simulink model "Project3_MODEL"  (R2023b)
settings: Solver=FixedStepAuto  StartTime=0.0  StopTime=765  FixedStep=0.001  RelTol=1e-3
values from neighbouring files (symbols this model uses):
  DriveData = [0 ... (first row only)    [initHighwayCycle.m]    (also in initUrbanCycle.m)
  mph2mps = 1600/3600    (= 0.444444444444)    [Project3_init.m]
  Time = (0:1:765)'    [initHighwayCycle.m]    (also in initUrbanCycle.m = (0:1:1369)')
undefined symbols (not defined in the file or in its folder): batData, carData, motorData
libraries: slpidlib x1
settings Model: Creator=anshu16  LastModifiedBy=turtl
settings OptimizationCC: ReuseModelBlockBuffer=off
settings DebuggingCC: UnconnectedInputMsg=warning  UnconnectedOutputMsg=warning  UnconnectedLineMsg=warning
settings ModelReferenceCC: EnableRefExpFcnMdlSchedulingChecks=on
settings SFSimCC: CustomCodeUndefinedFunction=UseInterfaceOnly

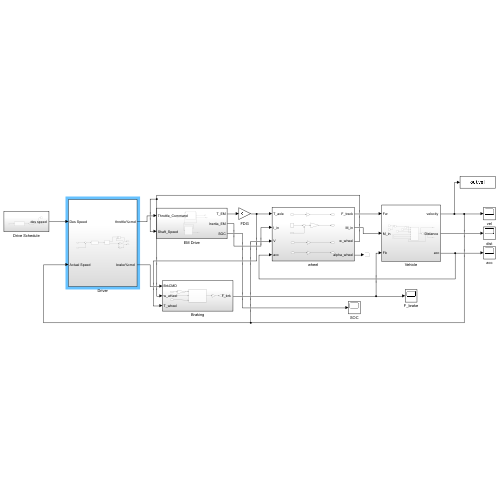
[thumbnail: Simulink's stored preview of the top-level diagram]
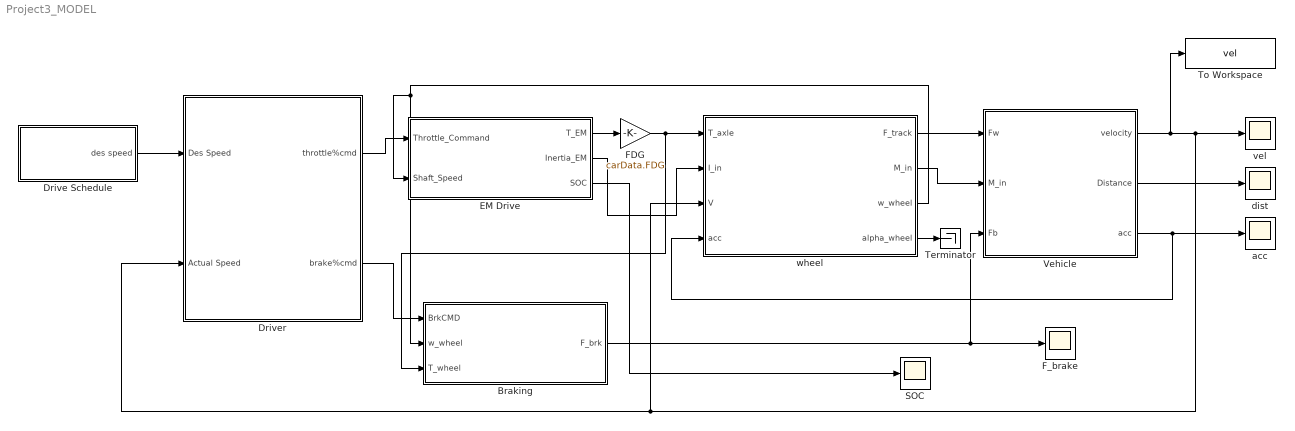
== system Project3_MODEL ==
  Braking : Subsystem
  Drive Schedule : Subsystem
  "Driver " : Subsystem
  EM Drive : Subsystem
  FDG : Gain  Gain=carData.FDG
  F_brake : Scope
  SOC : Scope
  Terminator : Terminator
  To Workspace : ToWorkspace  VariableName=vel  SaveFormat=Timeseries  SampleTime=-1
  Vehicle : Subsystem
  acc : Scope
  dist : Scope
  vel : Scope
  "wheel " : Subsystem
  wires:
  Drive Schedule/1("des speed ") -> "Driver "/1("Des Speed ")
  "Driver "/2("brake%cmd ") -> Braking/1("BrkCMD ")
  Braking/1("F_brk ") -> Vehicle/3("Fb "), F_brake/1
  Vehicle/3(acc) -> acc/1, "wheel "/4(acc)
  FDG/1 -> Braking/3(T_wheel), "wheel "/1(T_axle)
  EM Drive/2(Inertia_EM) -> "wheel "/2(I_in)
  "wheel "/2(M_in) -> Vehicle/2("M_in ")
  "wheel "/1(F_track) -> Vehicle/1("Fw ")
  Vehicle/2("Distance ") -> dist/1
  Vehicle/1("velocity ") -> To Workspace/1, vel/1, "wheel "/3(V), "Driver "/2(Actual Speed)
  "wheel "/4(alpha_wheel) -> Terminator/1
  "wheel "/3(w_wheel) -> Braking/2("w_wheel "), EM Drive/2(Shaft_Speed)
  "Driver "/1(throttle%cmd) -> EM Drive/1(Throttle_Command)
  EM Drive/3(SOC) -> SOC/1
  EM Drive/1(T_EM) -> FDG/1

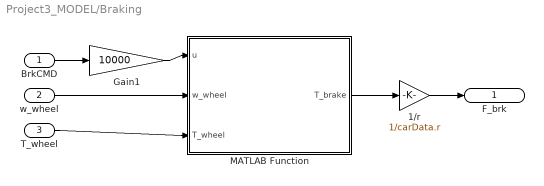
== system Project3_MODEL/Braking ==
  "BrkCMD " : Inport
  "w_wheel " : Inport  Port=2
  T_wheel : Inport  Port=3
  1/r : Gain  Gain=1/carData.r
  Gain1 : Gain  Gain=10000
  MATLAB Function : MATLAB Function  TreatAsAtomicUnit=on
  "F_brk " : Outport  VectorParamsAs1DForOutWhenUnconnected=off
  wires:
  "BrkCMD "/1 -> Gain1/1
  Gain1/1 -> MATLAB Function/1(u)
  MATLAB Function/1(T_brake) -> 1/r/1
  "w_wheel "/1 -> MATLAB Function/2(w_wheel)
  T_wheel/1 -> MATLAB Function/3(T_wheel)
  1/r/1 -> "F_brk "/1

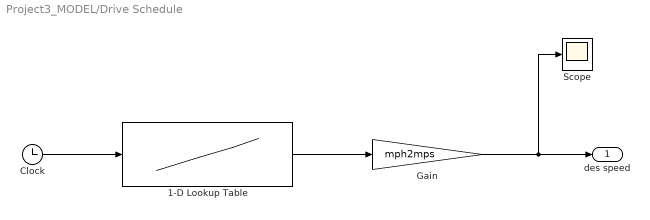
== system Project3_MODEL/Drive Schedule ==
  1-D Lookup Table : Lookup_n-D  NumberOfTableDimensions=1  BreakpointsForDimension1=Time  Table=DriveData  InternalRulePriority=Speed  RndMeth=Simplest
  Clock : Clock
  Gain : Gain  Gain=mph2mps
  Scope : Scope
  "des speed " : Outport  VectorParamsAs1DForOutWhenUnconnected=off
  wires:
  Clock/1 -> 1-D Lookup Table/1
  1-D Lookup Table/1 -> Gain/1
  Gain/1 -> "des speed "/1, Scope/1

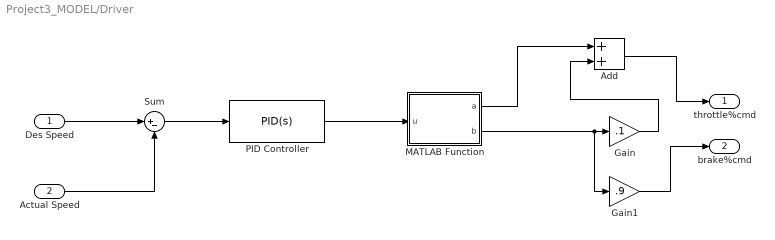
== system Project3_MODEL/Driver  ==
  "Des Speed " : Inport
  Actual Speed : Inport  Port=2
  Add : Sum
  Gain : Gain  Gain=.1
  Gain1 : Gain  Gain=.9
  MATLAB Function : MATLAB Function  TreatAsAtomicUnit=on
  PID Controller : slpidlib/PID Controller  Controller=PID  Form=Parallel  TimeDomain=Continuous-time  UseExternalTs=off  SampleTime=-1  IntegratorMethod=Forward Euler  FilterMethod=Forward Euler  ControllerParametersSource=internal  P=2.5  I=.1  UseKiTs=off  D=.5  N=100  UseFilter=on  TunerSelectOption=Transfer Function Based (PID Tuner App)  InitialConditionSource=internal  InitialConditionForIntegrator=0  InitialConditionForFilter=0  DifferentiatorICPrevScaledInput=0  ExternalReset=none  TrackingMode=off  Kt=1  LimitOutput=on  SatLimitsSource=internal  UpperSaturationLimit=1  LowerSaturationLimit=-1  LinearizeAsGain=off  AntiWindupMode=none  Kb=1  LimitIntegrator=off  UpperIntegratorSaturationLimit=inf  LowerIntegratorSaturationLimit=-inf  POutMin=[]  POutMax=[]  IOutMin=[]  IOutMax=[]  DOutMin=[]  DOutMax=[]  NOutMin=[]  NOutMax=[]  SumOutMin=[]  SumOutMax=[]  SaturationOutMin=[]  SaturationOutMax=[]  PParamMin=[]  PParamMax=[]  IParamMin=[]  IParamMax=[]  DParamMin=[]  DParamMax=[]  NParamMin=[]  NParamMax=[]  KbParamMin=[]  KbParamMax=[]  KtParamMin=[]  KtParamMax=[]  KbOutMin=[]  KbOutMax=[]  KtOutMin=[]  KtOutMax=[]  IntegratorOutMin=[]  IntegratorOutMax=[]  FilterOutMin=[]  FilterOutMax=[]  SumI1OutMin=[]  SumI1OutMax=[]  SumI2OutMin=[]  SumI2OutMax=[]  SumI3OutMin=[]  SumI3OutMax=[]  SumI4OutMin=[]  SumI4OutMax=[]  SumDOutMin=[]  SumDOutMax=[]  DifferentiatorOutMin=[]  DifferentiatorOutMax=[]  FilterDiffOutCoefMin=[]  FilterDiffOutCoefMax=[]  ReciprocalOutMin=[]  ReciprocalOutMax=[]  SumDenOutMin=[]  SumDenOutMax=[]  SumNumOutMin=[]  SumNumOutMax=[]  DivideOutMin=[]  DivideOutMax=[]  UdiffTsProdOutMin=[]  UdiffTsProdOutMax=[]  NTsProdOutMin=[]  NTsProdOutMax=[]  UintegralTsProdOutMin=[]  UintegralTsProdOutMax=[]  UngainTsProdOutMin=[]  UngainTsProdOutMax=[]  ClampingZeroOutDataTypeStr=Inherit: Inherit via back propagation  ClampingZeroOutMin=[]  ClampingZeroOutMax=[]  FilterDenConstantOutDataTypeStr=Inherit: Inherit via back propagation  FilterDenConstantOutMin=[]  FilterDenConstantOutMax=[]  PCopyOutDataTypeStr=Inherit: Inherit via back propagation  PCopyOutMin=[]  PCopyOutMax=[]  NCopyOutDataTypeStr=Inherit: Inherit via back propagation  NCopyOutMin=[]  NCopyOutMax=[]  IntegratorContinuousStateAttributes=''  IntegratorStateMustResolveToSignalObject=off  IntegratorRTWStateStorageClass=Auto  FilterContinuousStateAttributes=''  FilterStateMustResolveToSignalObject=off  FilterRTWStateStorageClass=Auto  ParallelPVariant=InternalParameters  IdealPVariant=Disabled  IVariant=InternalParameters  DVariant=InternalParameters  IntegratorVariant=Continuous  SatVariant=Enabled  AWVariant=Passthrough  PCopyVariant=Disabled  TRVariant=Disabled  FdbkBlocksVariant=Forward  IdealPFdbkVariant=Disabled  SatFdbkVariant=Disabled  DerivativeFilterVariant=ContFilter  NVariant=InternalParameters  NCopyVariant=Disabled  FilterICVariant=InternalICsFilter  IntegratorICVariant=InternalICs  ExternalResetVariant=Disabled  TRSumVariant=Passthrough  SumFdbkVariant=Disabled  SumVariant=Sum_PID  TsampFilterVariant=InternalTs  TsampNgainVariant=Passthrough  TsampIntegralVariant=Disabled_SignalSpec  ExternalSaturationOutDataTypeStr=Inherit: Same as second input
  Sum : Sum  Inputs=|+-
  throttle%cmd : Outport
  "brake%cmd " : Outport  Port=2
  wires:
  "Des Speed "/1 -> Sum/1
  Actual Speed/1 -> Sum/2
  Sum/1 -> PID Controller/1
  PID Controller/1 -> MATLAB Function/1(u)
  Gain/1 -> Add/2
  MATLAB Function/2(b) -> Gain/1, Gain1/1
  MATLAB Function/1(a) -> Add/1
  Add/1 -> throttle%cmd/1
  Gain1/1 -> "brake%cmd "/1

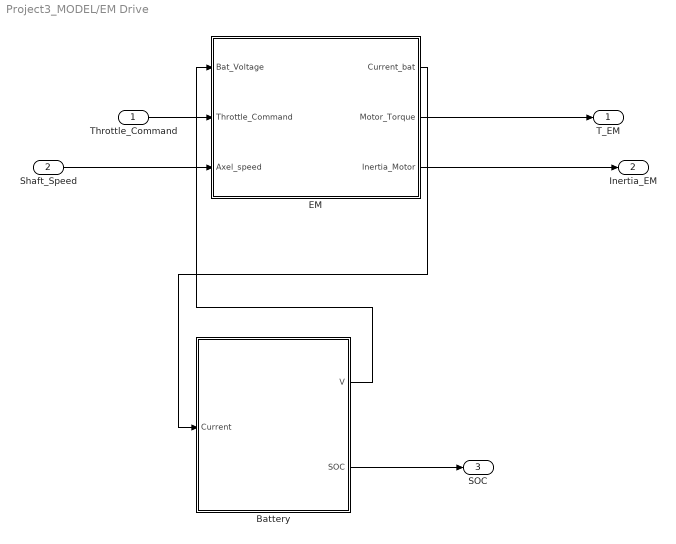
== system Project3_MODEL/EM Drive ==
  Throttle_Command : Inport
  Shaft_Speed : Inport  Port=2
  Battery : Subsystem
  EM : Subsystem
  T_EM : Outport
  Inertia_EM : Outport  Port=2
  SOC : Outport  Port=3
  wires:
  EM/1(Current_bat) -> Battery/1(Current)
  Throttle_Command/1 -> EM/2(Throttle_Command)
  Shaft_Speed/1 -> EM/3(Axel_speed)
  EM/2(Motor_Torque) -> T_EM/1
  EM/3(Inertia_Motor) -> Inertia_EM/1
  Battery/1(V) -> EM/1(Bat_Voltage)
  Battery/2(SOC) -> SOC/1

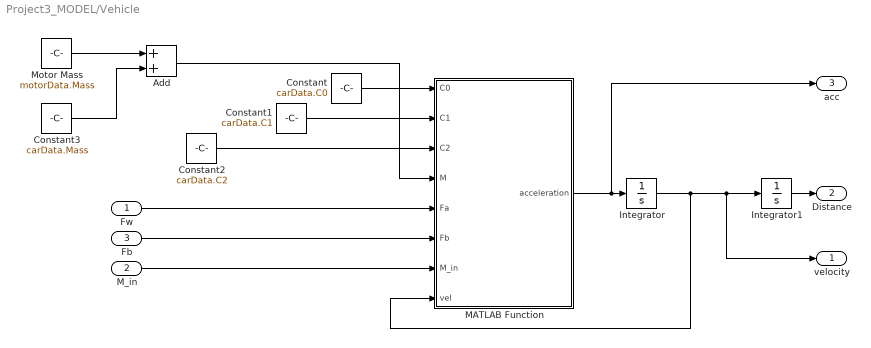
== system Project3_MODEL/Vehicle ==
  "Fw " : Inport
  "M_in " : Inport  Port=2
  "Fb " : Inport  Port=3
  Add : Sum
  Constant : Constant  Value=carData.C0
  Constant1 : Constant  Value=carData.C1
  Constant2 : Constant  Value=carData.C2
  Constant3 : Constant  Value=carData.Mass
  Integrator : Integrator  LimitOutput=on  LowerSaturationLimit=0
  Integrator1 : Integrator
  MATLAB Function : MATLAB Function  TreatAsAtomicUnit=on
  Motor Mass : Constant  Value=motorData.Mass
  "velocity " : Outport  VectorParamsAs1DForOutWhenUnconnected=off
  "Distance " : Outport  Port=2  VectorParamsAs1DForOutWhenUnconnected=off
  acc : Outport  Port=3
  wires:
  Constant1/1 -> MATLAB Function/2(C1)
  Constant/1 -> MATLAB Function/1(C0)
  MATLAB Function/1(acceleration) -> acc/1, Integrator/1
  Constant2/1 -> MATLAB Function/3(C2)
  Constant3/1 -> Add/2
  "Fw "/1 -> MATLAB Function/5(Fa)
  "Fb "/1 -> MATLAB Function/6(Fb)
  Integrator/1 -> MATLAB Function/8(vel), "velocity "/1, Integrator1/1
  Integrator1/1 -> "Distance "/1
  "M_in "/1 -> MATLAB Function/7(M_in)
  Motor Mass/1 -> Add/1
  Add/1 -> MATLAB Function/4(M)

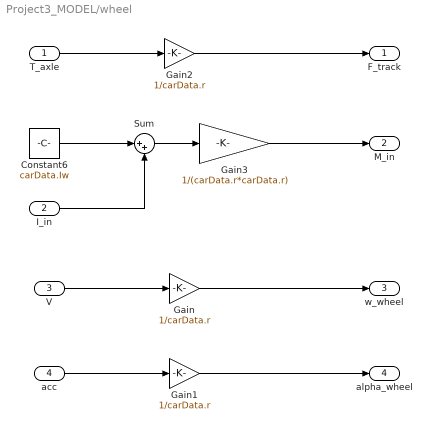
== system Project3_MODEL/wheel  ==
  T_axle : Inport
  I_in : Inport  Port=2
  V : Inport  Port=3
  acc : Inport  Port=4
  Constant6 : Constant  Value=carData.Iw
  Gain : Gain  Gain=1/carData.r
  Gain1 : Gain  Gain=1/carData.r
  Gain2 : Gain  Gain=1/carData.r
  Gain3 : Gain  Gain=1/(carData.r*carData.r)
  Sum : Sum  Inputs=|++
  F_track : Outport
  M_in : Outport  Port=2
  w_wheel : Outport  Port=3
  alpha_wheel : Outport  Port=4
  wires:
  Gain/1 -> w_wheel/1
  V/1 -> Gain/1
  acc/1 -> Gain1/1
  Gain1/1 -> alpha_wheel/1
  T_axle/1 -> Gain2/1
  Gain2/1 -> F_track/1
  Gain3/1 -> M_in/1
  Constant6/1 -> Sum/1
  I_in/1 -> Sum/2
  Sum/1 -> Gain3/1

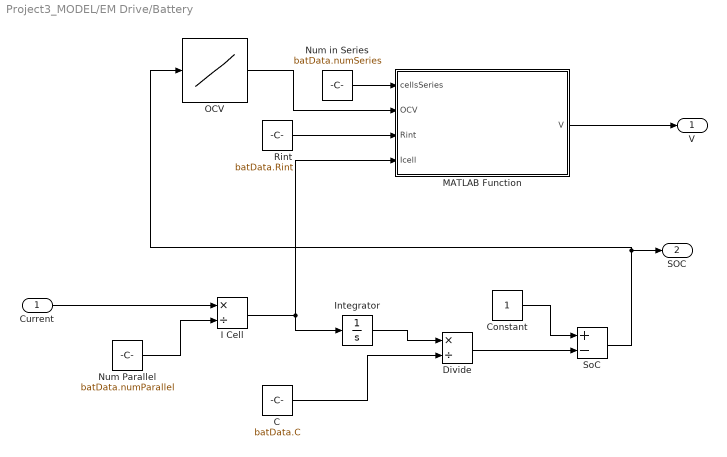
== system Project3_MODEL/EM Drive/Battery ==
  Current : Inport
  C : Constant  Value=batData.C
  Constant : Constant
  Divide : Product  Inputs=*/
  I Cell : Product  Inputs=*/
  Integrator : Integrator
  MATLAB Function : MATLAB Function  TreatAsAtomicUnit=on
  Num Parallel : Constant  Value=batData.numParallel
  Num in Series : Constant  Value=batData.numSeries
  OCV : Lookup_n-D  NumberOfTableDimensions=1  BreakpointsForDimension1=batData.SOC  BreakpointsForDimension2=[1:3]  Table=batData.OCV  InternalRulePriority=Speed  RndMeth=Simplest
  Rint : Constant  Value=batData.Rint
  SoC : Sum  Inputs=+-
  V : Outport
  SOC : Outport  Port=2
  wires:
  Num Parallel/1 -> I Cell/2
  I Cell/1 -> Integrator/1, MATLAB Function/4(Icell)
  C/1 -> Divide/2
  Integrator/1 -> Divide/1
  Divide/1 -> SoC/2
  SoC/1 -> SOC/1, OCV/1
  MATLAB Function/1(V) -> V/1
  OCV/1 -> MATLAB Function/2(OCV)
  Rint/1 -> MATLAB Function/3(Rint)
  Num in Series/1 -> MATLAB Function/1(cellsSeries)
  Constant/1 -> SoC/1
  Current/1 -> I Cell/1

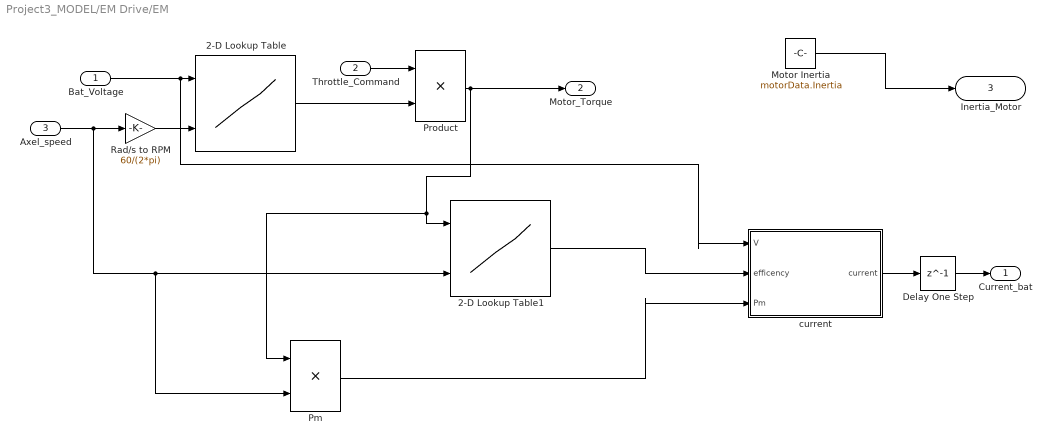
== system Project3_MODEL/EM Drive/EM ==
  Bat_Voltage : Inport
  Throttle_Command : Inport  Port=2
  Axel_speed : Inport  Port=3
  2-D Lookup Table : Lookup_n-D  BreakpointsForDimension1=motorData.vbus  BreakpointsForDimension2=motorData.rpm  Table=motorData.maxtorque  InternalRulePriority=Speed  RndMeth=Simplest
      settings: InputPortMap=u0,u1
  2-D Lookup Table1 : Lookup_n-D  BreakpointsForDimension1=motorData.eta_torque  BreakpointsForDimension2=motorData.eta_speed  Table=motorData.eta_val  InternalRulePriority=Speed  RndMeth=Simplest
      settings: InputPortMap=u0,u1
  Delay One Step : Delay  DelayLength=1
  Motor Inertia : Constant  Value=motorData.Inertia
  Pm : Product
  Product : Product
  Rad/s to RPM : Gain  Gain=60/(2*pi)
  current : MATLAB Function  TreatAsAtomicUnit=on
  Current_bat : Outport
  Motor_Torque : Outport  Port=2
  Inertia_Motor : Outport  Port=3
  wires:
  Axel_speed/1 -> Rad/s to RPM/1, 2-D Lookup Table1/2, Pm/2
  Bat_Voltage/1 -> current/1(V), 2-D Lookup Table/1
  2-D Lookup Table/1 -> Product/2
  Throttle_Command/1 -> Product/1
  Product/1 -> Pm/1, 2-D Lookup Table1/1, Motor_Torque/1
  Pm/1 -> current/3(Pm)
  2-D Lookup Table1/1 -> current/2(efficency)
  Motor Inertia/1 -> Inertia_Motor/1
  current/1(current) -> Delay One Step/1
  Rad/s to RPM/1 -> 2-D Lookup Table/2
  Delay One Step/1 -> Current_bat/1

== matlab function Project3_MODEL/Driver /MATLAB Function ==
  data: u input; a output; b output
function [a,b] = fcn(u)

if u>0
    acc=u;
    brk=0;
elseif u<0
    acc=0;
    brk=u;
else
    acc=0;
    brk=0;
end
a= acc;
b= brk;

== matlab function Project3_MODEL/Vehicle/MATLAB Function ==
  data: C0 input; acceleration output; C1 input; C2 input; M input; Fa input; Fb input; M_in input; vel input
function acceleration   = vehicle(C0,C1,C2,M,Fa,Fb,M_in, vel)

acceleration = (((Fa-Fb))-(C0+ C1*vel + C2*(vel)^2))/(M+M_in);

== matlab function Project3_MODEL/EM Drive/EM/current ==
  data: V input; current output; efficency input; Pm input
function current = fcn(V,efficency,Pm)

current = (Pm*efficency^(Pm/(abs(Pm)+.001)))/V;

== matlab function Project3_MODEL/EM Drive/Battery/MATLAB Function ==
  data: cellsSeries input; V output; OCV input; Rint input; Icell input
function V = fcn(cellsSeries,OCV,Rint,Icell)

V = cellsSeries*(OCV-Rint*Icell);

== matlab function Project3_MODEL/Braking/MATLAB Function ==
  data: u input; T_brake output; w_wheel input; T_wheel input
function T_brake = fcn(u,w_wheel,T_wheel)
%y = u*sign(w_wheel);
%y = 4*u * v/(abs(v)+0.0001);
%y = u;
Tb_cap = -u;
if w_wheel == 0
    T_brake = min(abs(T_wheel),Tb_cap)*w_wheel/(abs(w_wheel+.0001));
else
    T_brake =Tb_cap*w_wheel/(abs(w_wheel+.0001));
end
